simulink model "fengji"  (R2025a)
settings: Solver=VariableStepAuto  StartTime=0.0  StopTime=3  RelTol=1e-3
values from neighbouring files (symbols this model uses):
  A = pi * R^2    (= 6082.12337735)    [DFIG.m]    (also in Ref_and_Para.m)
  V = 0.9998    [Copy_2_of_wangce.m]    (also in Copy_2_of_wangceRef_and_Para.m; Copy_of_wangce.m; Copy_of_wangceRef_and_Para.m; DFIG.m)
undefined symbols (not defined in the file or in its folder): sigbuilder_block
libraries: slpidlib x6, spsabctodq0Lib x4, simulink x2, spsPLL3phLib x2, spsSVPWMGenerator2LevelLib x2, spsdq0toAlphaBetaZeroLib x2, spsUniversalBridgeLib x2, spsPower3phInstantaneousLib x1, spsSeriesRLCBranchLib x1, spsThreePhaseSeriesRLCBranchLib x1, spsThreePhaseVIMeasurementLib x1, spsThreePhaseSourceLib x1
settings Model: Creator=龙熠的本  LastModifiedBy=wz
settings SolverCC: AlgebraicLoopSolver=TrustRegion
settings DataIOCC: ReturnWorkspaceOutputs=off
settings DebuggingCC: UnconnectedInputMsg=warning  UnconnectedOutputMsg=warning  UnconnectedLineMsg=warning
settings ModelReferenceCC: EnableRefExpFcnMdlSchedulingChecks=on
settings RTWCC: GPUComputeCapability=3.5

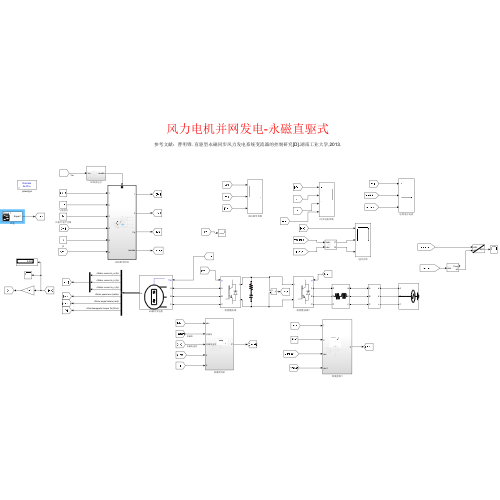
[thumbnail: Simulink's stored preview of the top-level diagram]
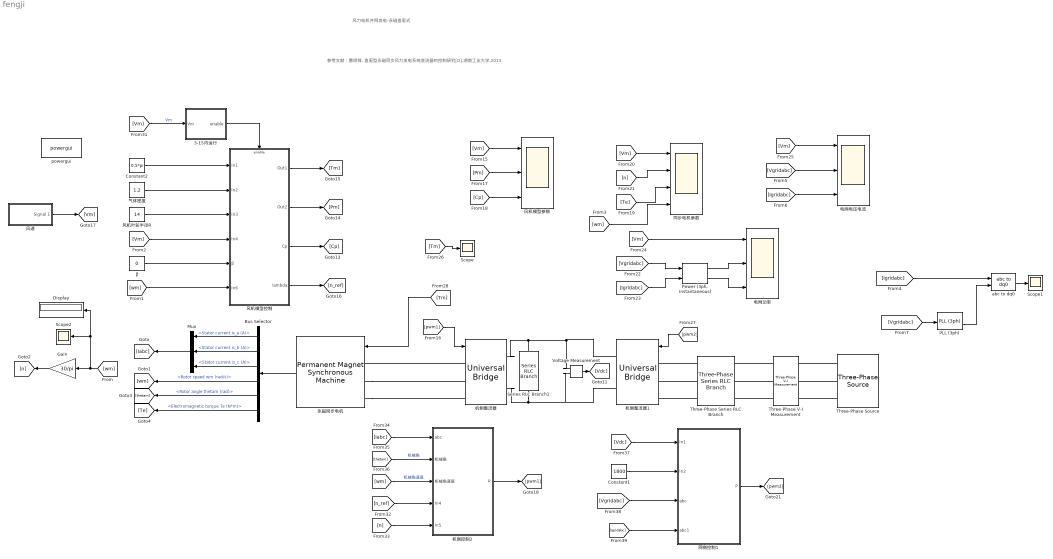
== system fengji ==
  note: 参考文献：曹明锋. 直驱型永磁同步风力发电系统变流器的控制研究[D].湖南工业大学,2013.
  note: 风力电机并网发电-永磁直驱式
  3-15内运行 : Subsystem
  Bus Selector : BusSelector  OutputSignals=Stator current is_a (A),Stator current is_b (A),Stator current is_c (A),Rotor speed wm (rad/s),Rotor angle thetam (rad),Electromagnetic torque Te (N*m)
  Constant1 : Constant  Value=1800
  Constant2 : Constant  Value=0.5*pi
  Display : Display
  Gain : Gain  Gain=30/pi
  Mux : Mux  Inputs=3
  PLL (3ph) : spsPLL3phLib/PLL (3ph)  Fmin=45  Par_Init=[0, 60]  ParK=[180, 3200, 1]  TcD=1e-4  MaxRateChangeFreq=12  FilterCutOffFreq=25  Ts=0  AGC=on
  "Power (3ph, Instantaneous)" : spsPower3phInstantaneousLib/Power (3ph, Instantaneous)
  Scope : Scope
      settings: ActiveDisplayYMinimum=-53568.9347809082  ActiveDisplayYMaximum=328.75957744243624  DataLoggingVariableName=ScopeData4
  Scope1 : Scope
      settings: ActiveDisplayYMinimum=-107.45342  ActiveDisplayYMaximum=357.3639
  Scope2 : Scope
      settings: DataLoggingVariableName=ScopeData9
  Series RLC Branch1 : spsSeriesRLCBranchLib/Series RLC Branch  LConnTagsString=__new0  RConnTagsString=__new0  BranchType=RC  Resistance=0.05  Inductance=1e-2  SetiL0=off  InitialCurrent=0  Capacitance=1e-3  Setx0=on  InitialVoltage=1800  Measurements=None
  Three-Phase Series RLC Branch : spsThreePhaseSeriesRLCBranchLib/Three-Phase Series RLC Branch  LConnTagsString=A|B|C  RConnTagsString=A|B|C  BranchType=RL  Resistance=0.05  Inductance=7e-3  Capacitance=1e-6  Measurements=None
  Three-Phase V-I Measurement : spsThreePhaseVIMeasurementLib/Three-Phase V-I Measurement  VoltageMeasurement=phase-to-ground  SetLabelV=on  LabelV=Vgridabc  Vpu=off  VpuLL=off  CurrentMeasurement=yes  SetLabelI=on  LabelI=Igridabc  Ipu=off  Pbase=100e6  Vbase=500e3  OutputType=Complex  PhasorSimulation=off  PSBequivalent=0
  Three-Phase Source : spsThreePhaseSourceLib/Three-Phase Source  InternalConnection=Yg  VoltagePhases=off  Voltage=690  PhaseAngle=0  Voltage_phases=[25e3 25e3 25e3]/sqrt(3)  PhaseAngles_phases=[0 -120 +120]  Frequency=50  NonIdealSource=off  SpecifyImpedance=off  Resistance=0.8929  Inductance=16.58e-3  ShortCircuitLevel=100e6  BaseVoltage=25e3  XRratio=7  BusType=swing  Pref=10e3  Qref=0  Prefabc=[10e3, 10e3, 10e3]  Qrefabc=[0, 0, 0]  Qmin=-inf  Qmax=inf
  Voltage Measurement : spsVoltageMeasurementLib/Voltage Measurement  PhasorSimulation=off  OutputType=Complex  PSBequivalent=0
  abc to dq0 : spsabctodq0Lib/abc to dq0  Alignment=90 degrees behind phase A axis
  powergui : sps_lib/powergui  Priority=1  SimulationMode=Discrete  SampleTime=2e-5  frequency=60  Iterations=50  frequencyindice=0  Pbase=100e6  ErrMax=1e-4  UnitsV=kV  UnitsW=MW  buscounter=0  FunctionMessages=off  echomessages=off  EnableUseOfTLC=off  CurrentSourceSwitches=off  DisableSnubberDevices=off  DisableRonSwitches=off  DisableVfSwitches=off  DisplayEquations=off  AutomaticDiscreteSolvers=off  SolverType=Tustin/Backward Euler (TBE)  Interpol=off  ExternalGateDelay=off  methode=off  Ts=100  x0status=blocks  SPID=on  SwTol=0  HookPort=off  NonlinearTolerance=1e-4  nMaxIteration=100  ContinueOnMaxIteration=off  RestoreLinks=warning  ResistiveCurrentMeasurement=off  Frange=[0:2:500]  Ylog=off  Xlog=on  ShowGrid=off  save=off  variable=ZData  structure=ScopeData3  ZoomFFT=off  StartTime=1.5  cycles=40  DisplayStyle=1  fundamental=50  FreqAxis=off  MaxFrequency=1000  frequencyindicesteady=1  RmsSteady=1  display=off
  β : Constant  Value=0
  同步电机参数 : Scope  NumInputPorts=4
      settings: ActiveDisplayYMinimum=7.5  ActiveDisplayYMaximum=12.5
  机侧控制2 : Subsystem
  机侧整流器 : spsUniversalBridgeLib/Universal Bridge  Arms=3  SnubberResistance=1e5  SnubberCapacitance=inf  Device=IGBT / Diodes  Ron=1e-3  Lon=0  ForwardVoltages="[  0  0  ]"  ForwardVoltage=0  GTOparameters=[ 10e-6 , 20e-6 ]  IGBTparameters=[ 1e-6 , 2e-6 ]  Measurements=None  Measurements_2=None  converterType=Rectifier
  机侧整流器1 : spsUniversalBridgeLib/Universal Bridge  Arms=3  SnubberResistance=1e5  SnubberCapacitance=inf  Device=IGBT / Diodes  Ron=1e-3  Lon=0  ForwardVoltages="[  0  0  ]"  ForwardVoltage=0  GTOparameters=[ 10e-6 , 20e-6 ]  IGBTparameters=[ 1e-6 , 2e-6 ]  Measurements=None  Measurements_2=None  converterType=Rectifier
  气体密度 : Constant  Value=1.2
  永磁同步电机 : spsPermanentMagnetSynchronousMachineLib/Permanent Magnet Synchronous Machine  NbPhases=3  FluxDistribution=Sinusoidal  RotorType=Round  MechanicalLoad=Torque Tm  PresetModel=No  ShowDetailedParameters=on  MeasurementBus=off  Resistance=0.025  Inductance=8.5e-3  dqInductances=[8.5e-3,8.5e-3]  La=0.0036  MachineConstant=Flux linkage established by magnets (V.s)  Flux=3.88889  VoltageCst=8464.3995  TorqueCst=70  Flat=120  Mechanical=[60 0.078 12]  PolePairs=4  InitialConditions=[0,0, 0,0]  InitialConditions5ph=[0 0 0 0 0 0]  RefAngle=90 degrees behind phase A axis (modified Park)  IterativeDiscreteModel=Trapezoidal non iterative  TsBlock=-1  TsPowergui=0
  电网功率 : Scope  NumInputPorts=3
      settings: ActiveDisplayYMinimum=2  ActiveDisplayYMaximum=22  DataLoggingVariableName=ScopeData2
  电网电压电流 : Scope  NumInputPorts=3
      settings: ActiveDisplayYMinimum=7.5  ActiveDisplayYMaximum=12.5  DataLoggingVariableName=ScopeData3
  网侧控制1 : Subsystem
  风机叶轮半径R : Constant  Value=14
  风机模型参数 : Scope  NumInputPorts=3
      settings: ActiveDisplayYMinimum=5.7582077  ActiveDisplayYMaximum=8.249088033333333
  风机模型控制 : Subsystem
  风速 : Subsystem  Tag=STV Subsys  LoadFcn=sigbuilder_block('load',[252.75 107.25 644.25 387.75 ]);  StartFcn=sigbuilder_block('start');  StopFcn=sigbuilder_block('stop');  ClipboardFcn=sigbuilder_block('clipboard');  mask(Sigbuilder block){tuvar=[0:10]}
      mask help: Simulink:masks:SigbuilderBlock_MD
      mask init:
      | if ~strcmp(get_param(bdroot(gcbh),'SimulationStatus'),'stopped') tuvar = sigbuilder_block('maskInit'); end
      settings: CopyFcn=sigbuilder_block('copy');  DeleteFcn=sigbuilder_block('delete');  ModelCloseFcn=sigbuilder_block('modelClose');  PreSaveFcn=sigbuilder_block('preSave');  PauseFcn=sigbuilder_block('pause');  ContinueFcn=sigbuilder_block('continue');  NameChangeFcn=sigbuilder_block('namechange');  OpenFcn=sigbuilder_block('open',[252.75 107.25 644.25 387.75 ]);  CloseFcn=sigbuilder_block('close');
      mask Display: plot(0, 0, 100, 100,[2, 2, 32, 32, 2], [68, 8, 8, 68, 68],[32, 2], [38, 38], [32, 19, 2],[53, 60, 44], [32, 17, 17, 2],[16, 16, 31, 31]);txt = getActiveGroup(gcbh);text(2, 100, txt,'verticalAlignment', 'top');
  wires:
  永磁同步电机/1 -> Bus Selector/1
  Bus Selector/2 -> Mux/2  "<Stator current is_b (A)>"
  Bus Selector/1 -> Mux/1  "<Stator current is_a (A)>"
  Bus Selector/3 -> Mux/3  "<Stator current is_c (A)>"
  Bus Selector/4 -> [wm]  "<Rotor speed wm (rad/s)>"
  Mux/1 -> [Iabc]
  Gain/1 -> [n]
  Bus Selector/5 -> [thetam]  "<Rotor angle thetam (rad)>"
  Bus Selector/6 -> [Te]  "<Electromagnetic torque Te (N*m)>"
  [wm] -> Display/1, Scope2/1, Gain/1
  [Tm] -> 永磁同步电机/1
  [pwm1] -> 机侧整流器/1
  [pwm2] -> 机侧整流器1/1
  [Vm] -> 风机模型参数/1
  [Pm] -> 风机模型参数/2
  [Cp] -> 风机模型参数/3
  [Vm] -> 同步电机参数/1
  [n] -> 同步电机参数/2
  [Te] -> 同步电机参数/3
  [Vgridabc] -> "Power (3ph, Instantaneous)"/1
  [Igridabc] -> "Power (3ph, Instantaneous)"/2
  "Power (3ph, Instantaneous)"/2 -> 电网功率/3
  "Power (3ph, Instantaneous)"/1 -> 电网功率/2
  [Vm] -> 电网功率/1
  [Vm] -> 电网电压电流/1
  [Vgridabc] -> 电网电压电流/2
  [Igridabc] -> 电网电压电流/3
  [Tm] -> Scope/1
  机侧控制2/1(P) -> [pwm1]
  [n] -> 机侧控制2/5(In5)
  [thetam] -> 机侧控制2/2(机械角)  "机械角"
  [Iabc] -> 机侧控制2/1(abc)
  [wm] -> 机侧控制2/3(机械角速度)  "机械角速度"
  [n_ref] -> 机侧控制2/4(In4)
  [Vgridabc] -> 网侧控制1/3(abc)
  网侧控制1/1(P) -> [pwm2]
  [Igridabc] -> 网侧控制1/4(abc1)
  Constant1/1 -> 网侧控制1/2(In2)
  [Vdc] -> 网侧控制1/1(In1)
  风速/1(Signal 1) -> [Vm]
  风机叶轮半径R/1 -> 风机模型控制/3(In3)
  Constant2/1 -> 风机模型控制/1(In1)
  风机模型控制/1(Out1) -> [Tm]
  风机模型控制/4(lambda) -> [n_ref]
  β/1 -> 风机模型控制/5(β)
  风机模型控制/3(Cp) -> [Cp]
  风机模型控制/2(Out2) -> [Pm]
  [wm] -> 风机模型控制/6(In6)
  气体密度/1 -> 风机模型控制/2(In2)
  3-15内运行/1(enable) -> 风机模型控制/Enable
  [Vm] -> 风机模型控制/4(In4)
  [Vm] -> 3-15内运行/1(Vm)  "Vm"
  Voltage Measurement/1 -> [Vdc]
  [wm] -> 同步电机参数/4
  [Vgridabc] -> PLL (3ph)/1
  [Igridabc] -> abc to dq0/1
  PLL (3ph)/2 -> abc to dq0/2
  abc to dq0/1 -> Scope1/1
  connections:
  机侧整流器/LConn1 -- 永磁同步电机/LConn1
  永磁同步电机/LConn2 -- 机侧整流器/LConn2
  永磁同步电机/LConn3 -- 机侧整流器/LConn3
  机侧整流器/RConn2 -- Voltage Measurement/LConn2 -- 机侧整流器1/RConn2 -- Series RLC Branch1/RConn1
  机侧整流器/RConn1 -- Series RLC Branch1/LConn1 -- 机侧整流器1/RConn1 -- Voltage Measurement/LConn1
  Three-Phase Series RLC Branch/LConn3 -- 机侧整流器1/LConn3
  Three-Phase Series RLC Branch/LConn2 -- 机侧整流器1/LConn2
  Three-Phase Series RLC Branch/LConn1 -- 机侧整流器1/LConn1
  Three-Phase V-I Measurement/LConn3 -- Three-Phase Series RLC Branch/RConn3
  Three-Phase V-I Measurement/LConn2 -- Three-Phase Series RLC Branch/RConn2
  Three-Phase V-I Measurement/LConn1 -- Three-Phase Series RLC Branch/RConn1
  Three-Phase Source/RConn3 -- Three-Phase V-I Measurement/RConn3
  Three-Phase Source/RConn2 -- Three-Phase V-I Measurement/RConn2
  Three-Phase Source/RConn1 -- Three-Phase V-I Measurement/RConn1

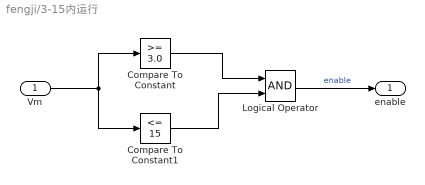
== system fengji/3-15内运行 ==
  Vm : Inport
  Compare To Constant : simulink/Logic and Bit Operations/Compare To Constant  relop=>=  const=3.0  OutDataTypeStr=boolean
  Compare To Constant1 : simulink/Logic and Bit Operations/Compare To Constant  relop=<=  const=15  OutDataTypeStr=boolean
  Logical Operator : Logic  AllPortsSameDT=off  OutDataTypeStr=boolean
  enable : Outport
  wires:
  Vm/1 -> Compare To Constant/1, Compare To Constant1/1
  Compare To Constant1/1 -> Logical Operator/2
  Logical Operator/1 -> enable/1  "enable"
  Compare To Constant/1 -> Logical Operator/1

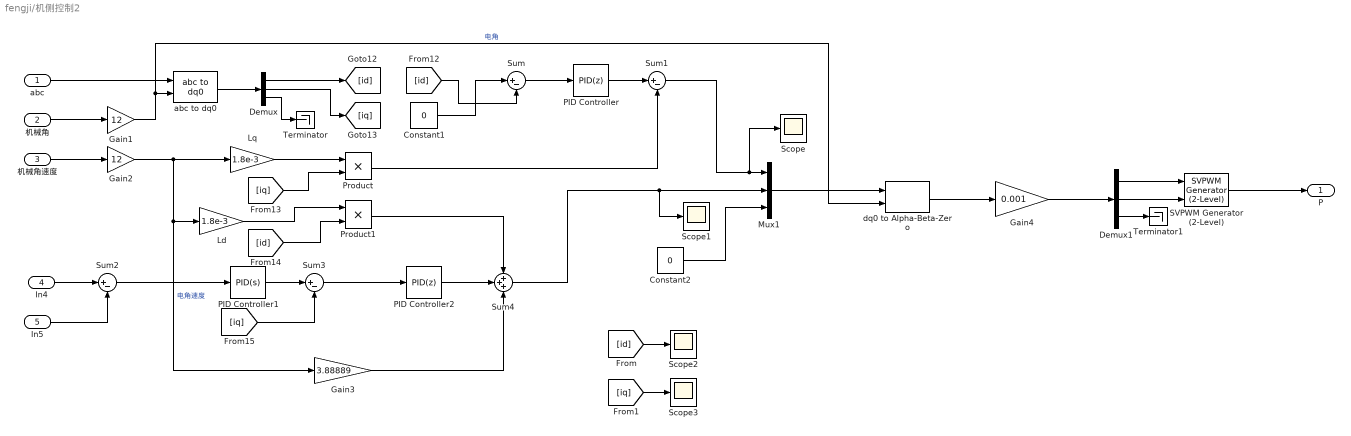
== system fengji/机侧控制2 ==
  abc : Inport
  机械角 : Inport  Port=2
  机械角速度 : Inport  Port=3
  In4 : Inport  Port=4
  In5 : Inport  Port=5
  Constant1 : Constant  Value=0
  Constant2 : Constant  Value=0
  Demux : Demux  Outputs=3
  Demux1 : Demux  Outputs=3
  Gain1 : Gain  Gain=12
  Gain2 : Gain  Gain=12
  Gain3 : Gain  Gain=3.88889
  Gain4 : Gain  Gain=0.001
  Ld : Gain  Gain=1.8e-3
  Lq : Gain  Gain=1.8e-3
  Mux1 : Mux  Inputs=3
  PID Controller : slpidlib/PID Controller  Controller=PID  Form=Parallel  TimeDomain=Discrete-time  UseExternalTs=off  SampleTime=-1  IntegratorMethod=Forward Euler  FilterMethod=Forward Euler  ControllerParametersSource=internal  P=1  I=12  UseKiTs=off  D=0  UseExternalDerivativeSource=off  N=100  UseFilter=on  TunerSelectOption=Transfer Function Based (PID Tuner App)  InitialConditionSource=internal  InitialConditionForIntegrator=0  InitialConditionForFilter=0  DifferentiatorICPrevScaledInput=0  ExternalReset=none  TrackingMode=off  Kt=1  LimitOutput=off  SatLimitsSource=internal  UpperSaturationLimit=inf  LowerSaturationLimit=-inf  LinearizeAsGain=on  AntiWindupMode=none  Kb=1  LimitIntegrator=off  UpperIntegratorSaturationLimit=inf  LowerIntegratorSaturationLimit=-inf  POutMin=[]  POutMax=[]  IOutMin=[]  IOutMax=[]  DOutMin=[]  DOutMax=[]  NOutMin=[]  NOutMax=[]  SumOutMin=[]  SumOutMax=[]  SaturationOutMin=[]  SaturationOutMax=[]  PParamMin=[]  PParamMax=[]  IParamMin=[]  IParamMax=[]  DParamMin=[]  DParamMax=[]  NParamMin=[]  NParamMax=[]  KbParamMin=[]  KbParamMax=[]  KtParamMin=[]  KtParamMax=[]  KbOutMin=[]  KbOutMax=[]  KtOutMin=[]  KtOutMax=[]  IntegratorOutMin=[]  IntegratorOutMax=[]  FilterOutMin=[]  FilterOutMax=[]  SumI1OutMin=[]  SumI1OutMax=[]  SumI2OutMin=[]  SumI2OutMax=[]  SumI3OutMin=[]  SumI3OutMax=[]  SumI4OutMin=[]  SumI4OutMax=[]  SumDOutMin=[]  SumDOutMax=[]  DifferentiatorOutMin=[]  DifferentiatorOutMax=[]  FilterDiffOutCoefMin=[]  FilterDiffOutCoefMax=[]  ReciprocalOutMin=[]  ReciprocalOutMax=[]  SumDenOutMin=[]  SumDenOutMax=[]  SumNumOutMin=[]  SumNumOutMax=[]  DivideOutMin=[]  DivideOutMax=[]  UdiffTsProdOutMin=[]  UdiffTsProdOutMax=[]  NTsProdOutMin=[]  NTsProdOutMax=[]  UintegralTsProdOutMin=[]  UintegralTsProdOutMax=[]  UngainTsProdOutMin=[]  UngainTsProdOutMax=[]  ClampingZeroOutDataTypeStr=Inherit: Inherit via back propagation  ClampingZeroOutMin=[]  ClampingZeroOutMax=[]  FilterDenConstantOutDataTypeStr=Inherit: Inherit via back propagation  FilterDenConstantOutMin=[]  FilterDenConstantOutMax=[]  PCopyOutDataTypeStr=Inherit: Inherit via back propagation  PCopyOutMin=[]  PCopyOutMax=[]  NCopyOutDataTypeStr=Inherit: Inherit via back propagation  NCopyOutMin=[]  NCopyOutMax=[]  IntegratorContinuousStateAttributes=''  IntegratorStateMustResolveToSignalObject=off  IntegratorRTWStateStorageClass=Auto  FilterContinuousStateAttributes=''  FilterStateMustResolveToSignalObject=off  FilterRTWStateStorageClass=Auto  ParallelPVariant=InternalParameters  IdealPVariant=Disabled  IVariant=InternalParameters  DVariant=InternalParameters  IntegratorVariant=Discrete  SatVariant=Disabled  AWVariant=Passthrough  PCopyVariant=Disabled  TRVariant=Disabled  FdbkBlocksVariant=Forward  IdealPFdbkVariant=Disabled  SatFdbkVariant=Disabled  DerivativeFilterVariant=ForwardEulerFilter  NVariant=InternalParameters  NCopyVariant=Disabled  FilterICVariant=InternalICsFilter  IntegratorICVariant=InternalICs  ExternalResetVariant=Disabled  TRSumVariant=Passthrough  SumFdbkVariant=Disabled  SumVariant=Sum_PID  TsampFilterVariant=InternalTs  TsampNgainVariant=Passthrough  TsampIntegralVariant=Disabled_SignalSpec  ExternalSaturationOutDataTypeStr=Inherit: Same as second input  DerivativeSourceVariant=ErrorSignal  PreIntVariant=InternalPreInt
  PID Controller1 : slpidlib/PID Controller  Controller=PID  Form=Parallel  TimeDomain=Continuous-time  UseExternalTs=off  SampleTime=-1  IntegratorMethod=Forward Euler  FilterMethod=Forward Euler  ControllerParametersSource=internal  P=10  I=220  UseKiTs=off  D=0  UseExternalDerivativeSource=off  N=100  UseFilter=on  TunerSelectOption=Transfer Function Based (PID Tuner App)  InitialConditionSource=internal  InitialConditionForIntegrator=0  InitialConditionForFilter=0  DifferentiatorICPrevScaledInput=0  ExternalReset=none  TrackingMode=off  Kt=1  LimitOutput=off  SatLimitsSource=internal  UpperSaturationLimit=inf  LowerSaturationLimit=-inf  LinearizeAsGain=on  AntiWindupMode=none  Kb=1  LimitIntegrator=off  UpperIntegratorSaturationLimit=inf  LowerIntegratorSaturationLimit=-inf  POutMin=[]  POutMax=[]  IOutMin=[]  IOutMax=[]  DOutMin=[]  DOutMax=[]  NOutMin=[]  NOutMax=[]  SumOutMin=[]  SumOutMax=[]  SaturationOutMin=[]  SaturationOutMax=[]  PParamMin=[]  PParamMax=[]  IParamMin=[]  IParamMax=[]  DParamMin=[]  DParamMax=[]  NParamMin=[]  NParamMax=[]  KbParamMin=[]  KbParamMax=[]  KtParamMin=[]  KtParamMax=[]  KbOutMin=[]  KbOutMax=[]  KtOutMin=[]  KtOutMax=[]  IntegratorOutMin=[]  IntegratorOutMax=[]  FilterOutMin=[]  FilterOutMax=[]  SumI1OutMin=[]  SumI1OutMax=[]  SumI2OutMin=[]  SumI2OutMax=[]  SumI3OutMin=[]  SumI3OutMax=[]  SumI4OutMin=[]  SumI4OutMax=[]  SumDOutMin=[]  SumDOutMax=[]  DifferentiatorOutMin=[]  DifferentiatorOutMax=[]  FilterDiffOutCoefMin=[]  FilterDiffOutCoefMax=[]  ReciprocalOutMin=[]  ReciprocalOutMax=[]  SumDenOutMin=[]  SumDenOutMax=[]  SumNumOutMin=[]  SumNumOutMax=[]  DivideOutMin=[]  DivideOutMax=[]  UdiffTsProdOutMin=[]  UdiffTsProdOutMax=[]  NTsProdOutMin=[]  NTsProdOutMax=[]  UintegralTsProdOutMin=[]  UintegralTsProdOutMax=[]  UngainTsProdOutMin=[]  UngainTsProdOutMax=[]  ClampingZeroOutDataTypeStr=Inherit: Inherit via back propagation  ClampingZeroOutMin=[]  ClampingZeroOutMax=[]  FilterDenConstantOutDataTypeStr=Inherit: Inherit via back propagation  FilterDenConstantOutMin=[]  FilterDenConstantOutMax=[]  PCopyOutDataTypeStr=Inherit: Inherit via back propagation  PCopyOutMin=[]  PCopyOutMax=[]  NCopyOutDataTypeStr=Inherit: Inherit via back propagation  NCopyOutMin=[]  NCopyOutMax=[]  IntegratorContinuousStateAttributes=''  IntegratorStateMustResolveToSignalObject=off  IntegratorRTWStateStorageClass=Auto  FilterContinuousStateAttributes=''  FilterStateMustResolveToSignalObject=off  FilterRTWStateStorageClass=Auto  ParallelPVariant=InternalParameters  IdealPVariant=Disabled  IVariant=InternalParameters  DVariant=InternalParameters  IntegratorVariant=Continuous  SatVariant=Disabled  AWVariant=Passthrough  PCopyVariant=Disabled  TRVariant=Disabled  FdbkBlocksVariant=Forward  IdealPFdbkVariant=Disabled  SatFdbkVariant=Disabled  DerivativeFilterVariant=ContFilter  NVariant=InternalParameters  NCopyVariant=Disabled  FilterICVariant=InternalICsFilter  IntegratorICVariant=InternalICs  ExternalResetVariant=Disabled  TRSumVariant=Passthrough  SumFdbkVariant=Disabled  SumVariant=Sum_PID  TsampFilterVariant=InternalTs  TsampNgainVariant=Passthrough  TsampIntegralVariant=Disabled_SignalSpec  ExternalSaturationOutDataTypeStr=Inherit: Same as second input  DerivativeSourceVariant=ErrorSignal  PreIntVariant=InternalPreInt
  PID Controller2 : slpidlib/PID Controller  Controller=PID  Form=Parallel  TimeDomain=Discrete-time  UseExternalTs=off  SampleTime=-1  IntegratorMethod=Forward Euler  FilterMethod=Forward Euler  ControllerParametersSource=internal  P=1  I=12  UseKiTs=off  D=0  UseExternalDerivativeSource=off  N=100  UseFilter=on  TunerSelectOption=Transfer Function Based (PID Tuner App)  InitialConditionSource=internal  InitialConditionForIntegrator=0  InitialConditionForFilter=0  DifferentiatorICPrevScaledInput=0  ExternalReset=none  TrackingMode=off  Kt=1  LimitOutput=off  SatLimitsSource=internal  UpperSaturationLimit=inf  LowerSaturationLimit=-inf  LinearizeAsGain=on  AntiWindupMode=none  Kb=1  LimitIntegrator=off  UpperIntegratorSaturationLimit=inf  LowerIntegratorSaturationLimit=-inf  POutMin=[]  POutMax=[]  IOutMin=[]  IOutMax=[]  DOutMin=[]  DOutMax=[]  NOutMin=[]  NOutMax=[]  SumOutMin=[]  SumOutMax=[]  SaturationOutMin=[]  SaturationOutMax=[]  PParamMin=[]  PParamMax=[]  IParamMin=[]  IParamMax=[]  DParamMin=[]  DParamMax=[]  NParamMin=[]  NParamMax=[]  KbParamMin=[]  KbParamMax=[]  KtParamMin=[]  KtParamMax=[]  KbOutMin=[]  KbOutMax=[]  KtOutMin=[]  KtOutMax=[]  IntegratorOutMin=[]  IntegratorOutMax=[]  FilterOutMin=[]  FilterOutMax=[]  SumI1OutMin=[]  SumI1OutMax=[]  SumI2OutMin=[]  SumI2OutMax=[]  SumI3OutMin=[]  SumI3OutMax=[]  SumI4OutMin=[]  SumI4OutMax=[]  SumDOutMin=[]  SumDOutMax=[]  DifferentiatorOutMin=[]  DifferentiatorOutMax=[]  FilterDiffOutCoefMin=[]  FilterDiffOutCoefMax=[]  ReciprocalOutMin=[]  ReciprocalOutMax=[]  SumDenOutMin=[]  SumDenOutMax=[]  SumNumOutMin=[]  SumNumOutMax=[]  DivideOutMin=[]  DivideOutMax=[]  UdiffTsProdOutMin=[]  UdiffTsProdOutMax=[]  NTsProdOutMin=[]  NTsProdOutMax=[]  UintegralTsProdOutMin=[]  UintegralTsProdOutMax=[]  UngainTsProdOutMin=[]  UngainTsProdOutMax=[]  ClampingZeroOutDataTypeStr=Inherit: Inherit via back propagation  ClampingZeroOutMin=[]  ClampingZeroOutMax=[]  FilterDenConstantOutDataTypeStr=Inherit: Inherit via back propagation  FilterDenConstantOutMin=[]  FilterDenConstantOutMax=[]  PCopyOutDataTypeStr=Inherit: Inherit via back propagation  PCopyOutMin=[]  PCopyOutMax=[]  NCopyOutDataTypeStr=Inherit: Inherit via back propagation  NCopyOutMin=[]  NCopyOutMax=[]  IntegratorContinuousStateAttributes=''  IntegratorStateMustResolveToSignalObject=off  IntegratorRTWStateStorageClass=Auto  FilterContinuousStateAttributes=''  FilterStateMustResolveToSignalObject=off  FilterRTWStateStorageClass=Auto  ParallelPVariant=InternalParameters  IdealPVariant=Disabled  IVariant=InternalParameters  DVariant=InternalParameters  IntegratorVariant=Discrete  SatVariant=Disabled  AWVariant=Passthrough  PCopyVariant=Disabled  TRVariant=Disabled  FdbkBlocksVariant=Forward  IdealPFdbkVariant=Disabled  SatFdbkVariant=Disabled  DerivativeFilterVariant=ForwardEulerFilter  NVariant=InternalParameters  NCopyVariant=Disabled  FilterICVariant=InternalICsFilter  IntegratorICVariant=InternalICs  ExternalResetVariant=Disabled  TRSumVariant=Passthrough  SumFdbkVariant=Disabled  SumVariant=Sum_PID  TsampFilterVariant=InternalTs  TsampNgainVariant=Passthrough  TsampIntegralVariant=Disabled_SignalSpec  ExternalSaturationOutDataTypeStr=Inherit: Same as second input  DerivativeSourceVariant=ErrorSignal  PreIntVariant=InternalPreInt
  Product : Product
  Product1 : Product
  SVPWM Generator (2-Level) : spsSVPWMGenerator2LevelLib/SVPWM Generator (2-Level)  InputType=alpha-beta components  SwitchingPattern=Pattern #1  Fc=3e3  ParUref=[0.8 -30 50]  Ts=0
  Scope{,1..3} (4 alike) : Scope
      Scope settings: ActiveDisplayYMinimum=-77.246328045068424  ActiveDisplayYMaximum=250.40861499738187  DataLoggingVariableName=ScopeData5
      Scope1 settings: ActiveDisplayYMinimum=51.447457334702889  ActiveDisplayYMaximum=486.78738885568737  DataLoggingVariableName=ScopeData6
      Scope2 settings: ActiveDisplayYMinimum=-70.304855275250532  ActiveDisplayYMaximum=40.582386040383945  DataLoggingVariableName=ScopeData7
      Scope3 settings: ActiveDisplayYMinimum=-769.28635625376307  ActiveDisplayYMaximum=430.28722806240035  DataLoggingVariableName=ScopeData8
  Sum{,1..3} (4 alike) : Sum  Inputs=|+-
  Sum4 : Sum  Inputs=+++
  Terminator : Terminator
  Terminator1 : Terminator
  abc to dq0 : spsabctodq0Lib/abc to dq0  Alignment=90 degrees behind phase A axis
  dq0 to Alpha-Beta-Zero : spsdq0toAlphaBetaZeroLib/dq0 to Alpha-Beta-Zero  Alignment=90 degrees behind phase A axis
  P : Outport
  wires:
  Sum4/1 -> Scope1/1, Mux1/2
  PID Controller1/1 -> Sum3/1
  Demux/2 -> [iq]
  Sum1/1 -> Scope/1, Mux1/1
  Demux/3 -> Terminator/1
  dq0 to Alpha-Beta-Zero/1 -> Gain4/1
  Demux/1 -> [id]
  SVPWM Generator (2-Level)/1 -> P/1
  [iq] -> Product/2
  Lq/1 -> Product/1
  [iq] -> Sum3/2
  [id] -> Product1/2
  Demux1/2 -> SVPWM Generator (2-Level)/2
  Sum/1 -> PID Controller/1
  Product/1 -> Sum1/2
  Gain1/1 -> dq0 to Alpha-Beta-Zero/2, abc to dq0/2  "电角"
  In4/1 -> Sum2/1
  Demux1/3 -> Terminator1/1
  Constant2/1 -> Mux1/3
  PID Controller2/1 -> Sum4/2
  abc to dq0/1 -> Demux/1
  Sum3/1 -> PID Controller2/1
  PID Controller/1 -> Sum1/1
  In5/1 -> Sum2/2
  Gain2/1 -> Gain3/1, Ld/1, Lq/1  "电角速度"
  Sum2/1 -> PID Controller1/1
  Ld/1 -> Product1/1
  Mux1/1 -> dq0 to Alpha-Beta-Zero/1
  机械角/1 -> Gain1/1
  机械角速度/1 -> Gain2/1
  Product1/1 -> Sum4/1
  Demux1/1 -> SVPWM Generator (2-Level)/1
  Gain3/1 -> Sum4/3
  Gain4/1 -> Demux1/1
  abc/1 -> abc to dq0/1
  Constant1/1 -> Sum/1
  [id] -> Sum/2
  [id] -> Scope2/1
  [iq] -> Scope3/1

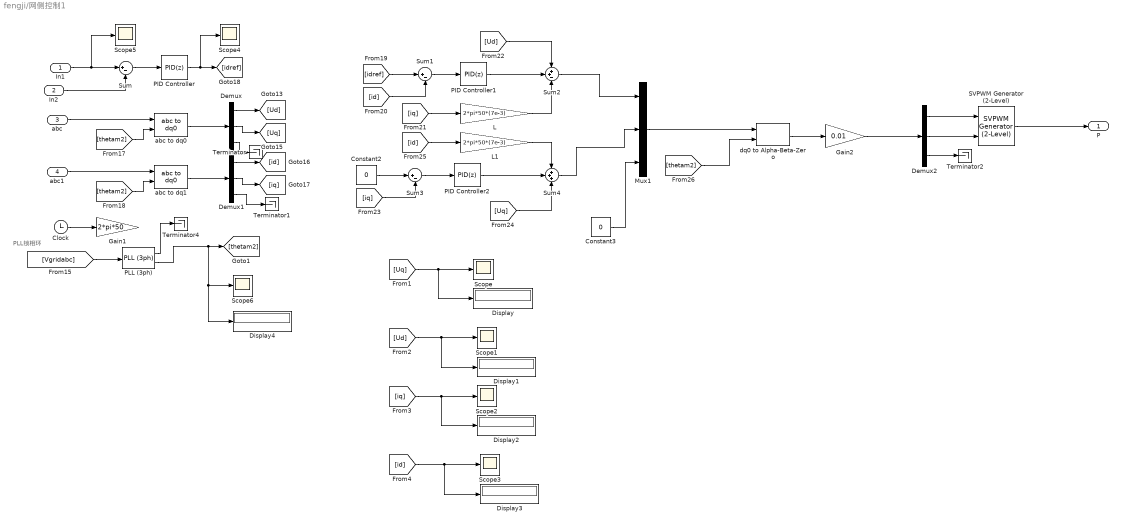
== system fengji/网侧控制1 ==
  note: PLL锁相环
  In1 : Inport
  In2 : Inport  Port=2
  abc : Inport  Port=3
  abc1 : Inport  Port=4
  Clock : Clock
  Constant2 : Constant  Value=0
  Constant3 : Constant  Value=0
  Demux : Demux  Outputs=3
  Demux1 : Demux  Outputs=3
  Demux2 : Demux  Outputs=3
  Display{,1..4} (5 alike) : Display
  Gain1 : Gain  Gain=2*pi*50
  Gain2 : Gain  Gain=0.01
  L : Gain  Gain=2*pi*50*(7e-3)
  L1 : Gain  Gain=2*pi*50*(7e-3)
  Mux1 : Mux  Inputs=3
  PID Controller : slpidlib/PID Controller  Controller=PID  Form=Parallel  TimeDomain=Discrete-time  UseExternalTs=off  SampleTime=-1  IntegratorMethod=Forward Euler  FilterMethod=Forward Euler  ControllerParametersSource=internal  P=1  I=10  UseKiTs=off  D=0  UseExternalDerivativeSource=off  N=100  UseFilter=on  TunerSelectOption=Transfer Function Based (PID Tuner App)  InitialConditionSource=internal  InitialConditionForIntegrator=0  InitialConditionForFilter=0  DifferentiatorICPrevScaledInput=0  ExternalReset=none  TrackingMode=off  Kt=1  LimitOutput=off  SatLimitsSource=internal  UpperSaturationLimit=inf  LowerSaturationLimit=-inf  LinearizeAsGain=on  AntiWindupMode=none  Kb=1  LimitIntegrator=off  UpperIntegratorSaturationLimit=inf  LowerIntegratorSaturationLimit=-inf  POutMin=[]  POutMax=[]  IOutMin=[]  IOutMax=[]  DOutMin=[]  DOutMax=[]  NOutMin=[]  NOutMax=[]  SumOutMin=[]  SumOutMax=[]  SaturationOutMin=[]  SaturationOutMax=[]  PParamMin=[]  PParamMax=[]  IParamMin=[]  IParamMax=[]  DParamMin=[]  DParamMax=[]  NParamMin=[]  NParamMax=[]  KbParamMin=[]  KbParamMax=[]  KtParamMin=[]  KtParamMax=[]  KbOutMin=[]  KbOutMax=[]  KtOutMin=[]  KtOutMax=[]  IntegratorOutMin=[]  IntegratorOutMax=[]  FilterOutMin=[]  FilterOutMax=[]  SumI1OutMin=[]  SumI1OutMax=[]  SumI2OutMin=[]  SumI2OutMax=[]  SumI3OutMin=[]  SumI3OutMax=[]  SumI4OutMin=[]  SumI4OutMax=[]  SumDOutMin=[]  SumDOutMax=[]  DifferentiatorOutMin=[]  DifferentiatorOutMax=[]  FilterDiffOutCoefMin=[]  FilterDiffOutCoefMax=[]  ReciprocalOutMin=[]  ReciprocalOutMax=[]  SumDenOutMin=[]  SumDenOutMax=[]  SumNumOutMin=[]  SumNumOutMax=[]  DivideOutMin=[]  DivideOutMax=[]  UdiffTsProdOutMin=[]  UdiffTsProdOutMax=[]  NTsProdOutMin=[]  NTsProdOutMax=[]  UintegralTsProdOutMin=[]  UintegralTsProdOutMax=[]  UngainTsProdOutMin=[]  UngainTsProdOutMax=[]  ClampingZeroOutDataTypeStr=Inherit: Inherit via back propagation  ClampingZeroOutMin=[]  ClampingZeroOutMax=[]  FilterDenConstantOutDataTypeStr=Inherit: Inherit via back propagation  FilterDenConstantOutMin=[]  FilterDenConstantOutMax=[]  PCopyOutDataTypeStr=Inherit: Inherit via back propagation  PCopyOutMin=[]  PCopyOutMax=[]  NCopyOutDataTypeStr=Inherit: Inherit via back propagation  NCopyOutMin=[]  NCopyOutMax=[]  IntegratorContinuousStateAttributes=''  IntegratorStateMustResolveToSignalObject=off  IntegratorRTWStateStorageClass=Auto  FilterContinuousStateAttributes=''  FilterStateMustResolveToSignalObject=off  FilterRTWStateStorageClass=Auto  ParallelPVariant=InternalParameters  IdealPVariant=Disabled  IVariant=InternalParameters  DVariant=InternalParameters  IntegratorVariant=Discrete  SatVariant=Disabled  AWVariant=Passthrough  PCopyVariant=Disabled  TRVariant=Disabled  FdbkBlocksVariant=Forward  IdealPFdbkVariant=Disabled  SatFdbkVariant=Disabled  DerivativeFilterVariant=ForwardEulerFilter  NVariant=InternalParameters  NCopyVariant=Disabled  FilterICVariant=InternalICsFilter  IntegratorICVariant=InternalICs  ExternalResetVariant=Disabled  TRSumVariant=Passthrough  SumFdbkVariant=Disabled  SumVariant=Sum_PID  TsampFilterVariant=InternalTs  TsampNgainVariant=Passthrough  TsampIntegralVariant=Disabled_SignalSpec  ExternalSaturationOutDataTypeStr=Inherit: Same as second input  DerivativeSourceVariant=ErrorSignal  PreIntVariant=InternalPreInt
  PID Controller1 : slpidlib/PID Controller  Controller=PID  Form=Parallel  TimeDomain=Discrete-time  UseExternalTs=off  SampleTime=-1  IntegratorMethod=Forward Euler  FilterMethod=Forward Euler  ControllerParametersSource=internal  P=1  I=15  UseKiTs=off  D=0  UseExternalDerivativeSource=off  N=100  UseFilter=on  TunerSelectOption=Transfer Function Based (PID Tuner App)  InitialConditionSource=internal  InitialConditionForIntegrator=0  InitialConditionForFilter=0  DifferentiatorICPrevScaledInput=0  ExternalReset=none  TrackingMode=off  Kt=1  LimitOutput=off  SatLimitsSource=internal  UpperSaturationLimit=inf  LowerSaturationLimit=-inf  LinearizeAsGain=on  AntiWindupMode=none  Kb=1  LimitIntegrator=off  UpperIntegratorSaturationLimit=inf  LowerIntegratorSaturationLimit=-inf  POutMin=[]  POutMax=[]  IOutMin=[]  IOutMax=[]  DOutMin=[]  DOutMax=[]  NOutMin=[]  NOutMax=[]  SumOutMin=[]  SumOutMax=[]  SaturationOutMin=[]  SaturationOutMax=[]  PParamMin=[]  PParamMax=[]  IParamMin=[]  IParamMax=[]  DParamMin=[]  DParamMax=[]  NParamMin=[]  NParamMax=[]  KbParamMin=[]  KbParamMax=[]  KtParamMin=[]  KtParamMax=[]  KbOutMin=[]  KbOutMax=[]  KtOutMin=[]  KtOutMax=[]  IntegratorOutMin=[]  IntegratorOutMax=[]  FilterOutMin=[]  FilterOutMax=[]  SumI1OutMin=[]  SumI1OutMax=[]  SumI2OutMin=[]  SumI2OutMax=[]  SumI3OutMin=[]  SumI3OutMax=[]  SumI4OutMin=[]  SumI4OutMax=[]  SumDOutMin=[]  SumDOutMax=[]  DifferentiatorOutMin=[]  DifferentiatorOutMax=[]  FilterDiffOutCoefMin=[]  FilterDiffOutCoefMax=[]  ReciprocalOutMin=[]  ReciprocalOutMax=[]  SumDenOutMin=[]  SumDenOutMax=[]  SumNumOutMin=[]  SumNumOutMax=[]  DivideOutMin=[]  DivideOutMax=[]  UdiffTsProdOutMin=[]  UdiffTsProdOutMax=[]  NTsProdOutMin=[]  NTsProdOutMax=[]  UintegralTsProdOutMin=[]  UintegralTsProdOutMax=[]  UngainTsProdOutMin=[]  UngainTsProdOutMax=[]  ClampingZeroOutDataTypeStr=Inherit: Inherit via back propagation  ClampingZeroOutMin=[]  ClampingZeroOutMax=[]  FilterDenConstantOutDataTypeStr=Inherit: Inherit via back propagation  FilterDenConstantOutMin=[]  FilterDenConstantOutMax=[]  PCopyOutDataTypeStr=Inherit: Inherit via back propagation  PCopyOutMin=[]  PCopyOutMax=[]  NCopyOutDataTypeStr=Inherit: Inherit via back propagation  NCopyOutMin=[]  NCopyOutMax=[]  IntegratorContinuousStateAttributes=''  IntegratorStateMustResolveToSignalObject=off  IntegratorRTWStateStorageClass=Auto  FilterContinuousStateAttributes=''  FilterStateMustResolveToSignalObject=off  FilterRTWStateStorageClass=Auto  ParallelPVariant=InternalParameters  IdealPVariant=Disabled  IVariant=InternalParameters  DVariant=InternalParameters  IntegratorVariant=Discrete  SatVariant=Disabled  AWVariant=Passthrough  PCopyVariant=Disabled  TRVariant=Disabled  FdbkBlocksVariant=Forward  IdealPFdbkVariant=Disabled  SatFdbkVariant=Disabled  DerivativeFilterVariant=ForwardEulerFilter  NVariant=InternalParameters  NCopyVariant=Disabled  FilterICVariant=InternalICsFilter  IntegratorICVariant=InternalICs  ExternalResetVariant=Disabled  TRSumVariant=Passthrough  SumFdbkVariant=Disabled  SumVariant=Sum_PID  TsampFilterVariant=InternalTs  TsampNgainVariant=Passthrough  TsampIntegralVariant=Disabled_SignalSpec  ExternalSaturationOutDataTypeStr=Inherit: Same as second input  DerivativeSourceVariant=ErrorSignal  PreIntVariant=InternalPreInt
  PID Controller2 : slpidlib/PID Controller  Controller=PID  Form=Parallel  TimeDomain=Discrete-time  UseExternalTs=off  SampleTime=-1  IntegratorMethod=Forward Euler  FilterMethod=Forward Euler  ControllerParametersSource=internal  P=1  I=15  UseKiTs=off  D=0  UseExternalDerivativeSource=off  N=100  UseFilter=on  TunerSelectOption=Transfer Function Based (PID Tuner App)  InitialConditionSource=internal  InitialConditionForIntegrator=0  InitialConditionForFilter=0  DifferentiatorICPrevScaledInput=0  ExternalReset=none  TrackingMode=off  Kt=1  LimitOutput=off  SatLimitsSource=internal  UpperSaturationLimit=inf  LowerSaturationLimit=-inf  LinearizeAsGain=on  AntiWindupMode=none  Kb=1  LimitIntegrator=off  UpperIntegratorSaturationLimit=inf  LowerIntegratorSaturationLimit=-inf  POutMin=[]  POutMax=[]  IOutMin=[]  IOutMax=[]  DOutMin=[]  DOutMax=[]  NOutMin=[]  NOutMax=[]  SumOutMin=[]  SumOutMax=[]  SaturationOutMin=[]  SaturationOutMax=[]  PParamMin=[]  PParamMax=[]  IParamMin=[]  IParamMax=[]  DParamMin=[]  DParamMax=[]  NParamMin=[]  NParamMax=[]  KbParamMin=[]  KbParamMax=[]  KtParamMin=[]  KtParamMax=[]  KbOutMin=[]  KbOutMax=[]  KtOutMin=[]  KtOutMax=[]  IntegratorOutMin=[]  IntegratorOutMax=[]  FilterOutMin=[]  FilterOutMax=[]  SumI1OutMin=[]  SumI1OutMax=[]  SumI2OutMin=[]  SumI2OutMax=[]  SumI3OutMin=[]  SumI3OutMax=[]  SumI4OutMin=[]  SumI4OutMax=[]  SumDOutMin=[]  SumDOutMax=[]  DifferentiatorOutMin=[]  DifferentiatorOutMax=[]  FilterDiffOutCoefMin=[]  FilterDiffOutCoefMax=[]  ReciprocalOutMin=[]  ReciprocalOutMax=[]  SumDenOutMin=[]  SumDenOutMax=[]  SumNumOutMin=[]  SumNumOutMax=[]  DivideOutMin=[]  DivideOutMax=[]  UdiffTsProdOutMin=[]  UdiffTsProdOutMax=[]  NTsProdOutMin=[]  NTsProdOutMax=[]  UintegralTsProdOutMin=[]  UintegralTsProdOutMax=[]  UngainTsProdOutMin=[]  UngainTsProdOutMax=[]  ClampingZeroOutDataTypeStr=Inherit: Inherit via back propagation  ClampingZeroOutMin=[]  ClampingZeroOutMax=[]  FilterDenConstantOutDataTypeStr=Inherit: Inherit via back propagation  FilterDenConstantOutMin=[]  FilterDenConstantOutMax=[]  PCopyOutDataTypeStr=Inherit: Inherit via back propagation  PCopyOutMin=[]  PCopyOutMax=[]  NCopyOutDataTypeStr=Inherit: Inherit via back propagation  NCopyOutMin=[]  NCopyOutMax=[]  IntegratorContinuousStateAttributes=''  IntegratorStateMustResolveToSignalObject=off  IntegratorRTWStateStorageClass=Auto  FilterContinuousStateAttributes=''  FilterStateMustResolveToSignalObject=off  FilterRTWStateStorageClass=Auto  ParallelPVariant=InternalParameters  IdealPVariant=Disabled  IVariant=InternalParameters  DVariant=InternalParameters  IntegratorVariant=Discrete  SatVariant=Disabled  AWVariant=Passthrough  PCopyVariant=Disabled  TRVariant=Disabled  FdbkBlocksVariant=Forward  IdealPFdbkVariant=Disabled  SatFdbkVariant=Disabled  DerivativeFilterVariant=ForwardEulerFilter  NVariant=InternalParameters  NCopyVariant=Disabled  FilterICVariant=InternalICsFilter  IntegratorICVariant=InternalICs  ExternalResetVariant=Disabled  TRSumVariant=Passthrough  SumFdbkVariant=Disabled  SumVariant=Sum_PID  TsampFilterVariant=InternalTs  TsampNgainVariant=Passthrough  TsampIntegralVariant=Disabled_SignalSpec  ExternalSaturationOutDataTypeStr=Inherit: Same as second input  DerivativeSourceVariant=ErrorSignal  PreIntVariant=InternalPreInt
  PLL (3ph) : spsPLL3phLib/PLL (3ph)  Fmin=45  Par_Init=[0, 50]  ParK=[180, 3200, 1]  TcD=1e-4  MaxRateChangeFreq=12  FilterCutOffFreq=25  Ts=0  AGC=on
  SVPWM Generator (2-Level) : spsSVPWMGenerator2LevelLib/SVPWM Generator (2-Level)  InputType=alpha-beta components  SwitchingPattern=Pattern #1  Fc=3000  ParUref=[0.8 -30 50]  Ts=0
  Scope{,1..6} (7 alike) : Scope
      Scope settings: ActiveDisplayYMinimum=-4.34345536667807  ActiveDisplayYMaximum=3.6929558988105935  DataLoggingVariableName=ScopeData10
      Scope1 settings: ActiveDisplayYMinimum=563.37013006275  ActiveDisplayYMaximum=563.38403092650674  DataLoggingVariableName=ScopeData11
      Scope2 settings: ActiveDisplayYMinimum=-203.1682368264394  ActiveDisplayYMaximum=403.27940369592733  DataLoggingVariableName=ScopeData12
      Scope3 settings: ActiveDisplayYMinimum=-661.11803433014575  ActiveDisplayYMaximum=608.254667322305  DataLoggingVariableName=ScopeData13
      Scope4 settings: ActiveDisplayYMinimum=-1055.4396971227802  ActiveDisplayYMaximum=1429.5603673337337  DataLoggingVariableName=ScopeData14
      Scope5 settings: ActiveDisplayYMinimum=806.5413726592958  ActiveDisplayYMaximum=3282.30252742951  DataLoggingVariableName=ScopeData15
      Scope6 settings: ActiveDisplayYMinimum=-0.785398163397448  ActiveDisplayYMaximum=7.0685834705770336  DataLoggingVariableName=ScopeData16
  Sum : Sum  Inputs=|+-
  Sum1 : Sum  Inputs=|+-
  Sum2 : Sum  Inputs=++-
  Sum3 : Sum  Inputs=|+-
  Sum4 : Sum  Inputs=+++
  Terminator{,1..2,4} (4 alike) : Terminator
  abc to dq0 : spsabctodq0Lib/abc to dq0  Alignment=90 degrees behind phase A axis
  abc to dq1 : spsabctodq0Lib/abc to dq0  Alignment=90 degrees behind phase A axis
  dq0 to Alpha-Beta-Zero : spsdq0toAlphaBetaZeroLib/dq0 to Alpha-Beta-Zero  Alignment=90 degrees behind phase A axis
  P : Outport
  wires:
  [thetam2] -> abc to dq1/2
  [id] -> Sum1/2
  abc to dq1/1 -> Demux1/1
  PID Controller/1 -> Scope4/1, [idref]
  Gain2/1 -> Demux2/1
  [thetam2] -> abc to dq0/2
  abc1/1 -> abc to dq1/1
  Sum4/1 -> Mux1/2
  [iq] -> Sum3/2
  abc to dq0/1 -> Demux/1
  Demux1/3 -> Terminator1/1
  Demux1/2 -> [iq]
  Constant2/1 -> Sum3/1
  Demux1/1 -> [id]
  PID Controller2/1 -> Sum4/2
  Demux2/1 -> SVPWM Generator (2-Level)/1
  L1/1 -> Sum4/1
  Demux/1 -> [Ud]
  SVPWM Generator (2-Level)/1 -> P/1
  Demux/3 -> Terminator/1
  [Vgridabc] -> PLL (3ph)/1
  Demux2/2 -> SVPWM Generator (2-Level)/2
  Demux/2 -> [Uq]
  PID Controller1/1 -> Sum2/2
  Sum1/1 -> PID Controller1/1
  L/1 -> Sum2/3
  Clock/1 -> Gain1/1
  Sum3/1 -> PID Controller2/1
  Sum/1 -> PID Controller/1
  Demux2/3 -> Terminator2/1
  Mux1/1 -> dq0 to Alpha-Beta-Zero/1
  dq0 to Alpha-Beta-Zero/1 -> Gain2/1
  [Ud] -> Sum2/1
  [iq] -> L/1
  In2/1 -> Sum/2
  [thetam2] -> dq0 to Alpha-Beta-Zero/2
  abc/1 -> abc to dq0/1
  [Uq] -> Sum4/3
  [idref] -> Sum1/1
  [id] -> L1/1
  In1/1 -> Scope5/1, Sum/1
  PLL (3ph)/2 -> Display4/1, Scope6/1, [thetam2]
  Constant3/1 -> Mux1/3
  Sum2/1 -> Mux1/1
  [Uq] -> Display/1, Scope/1
  [Ud] -> Scope1/1, Display1/1
  [id] -> Display3/1, Scope3/1
  [iq] -> Scope2/1, Display2/1
  PLL (3ph)/1 -> Terminator4/1

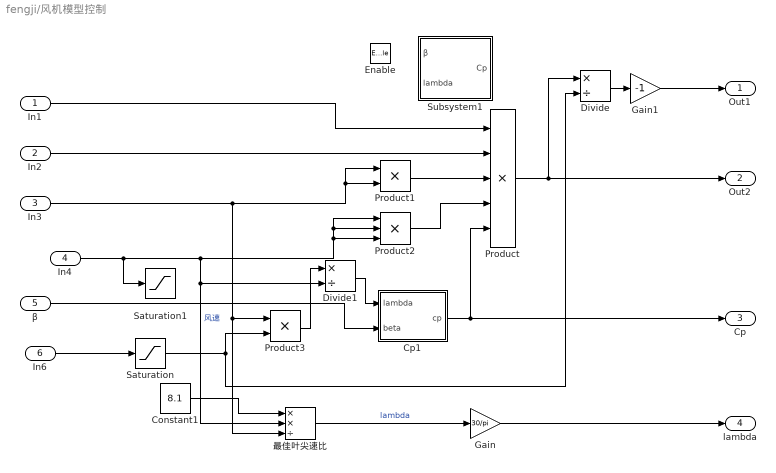
== system fengji/风机模型控制 ==
  In1 : Inport
  In2 : Inport  Port=2
  In3 : Inport  Port=3
  In4 : Inport  Port=4
  β : Inport  Port=5
  In6 : Inport  Port=6
  Enable : EnablePort
  Constant1 : Constant  Value=8.1
  Cp1 : Subsystem
  Divide : Product  Inputs=*/
  Divide1 : Product  Inputs=*/
  Gain : Gain  Gain=30/pi
  Gain1 : Gain  Gain=-1
  Product : Product  Inputs=5
  Product1 : Product
  Product2 : Product  Inputs=3
  Product3 : Product
  Saturation : Saturate  UpperLimit=1e6  LowerLimit=1e-6
  Saturation1 : Saturate  UpperLimit=1e6  LowerLimit=1e-6
  Subsystem1 : Subsystem
  最佳叶尖速比 : Product  Inputs=**/
  Out1 : Outport
  Out2 : Outport  Port=2
  Cp : Outport  Port=3
  lambda : Outport  Port=4
  wires:
  Product2/1 -> Product/4
  Divide/1 -> Gain1/1
  In3/1 -> Product3/1, 最佳叶尖速比/3, Product1/1, Product1/2
  Saturation/1 -> Divide/2, Product3/2
  Cp1/1(cp) -> Cp/1, Product/5
  Constant1/1 -> 最佳叶尖速比/1
  Product/1 -> Out2/1, Divide/1
  Product1/1 -> Product/3
  In4/1 -> Saturation1/1, Divide1/2, 最佳叶尖速比/2, Product2/3, Product2/2, Product2/1  "风速"
  In1/1 -> Product/1
  In6/1 -> Saturation/1
  Gain1/1 -> Out1/1
  In2/1 -> Product/2
  最佳叶尖速比/1 -> Gain/1  "lambda"
  β/1 -> Cp1/2(beta)
  Product3/1 -> Divide1/1
  Divide1/1 -> Cp1/1(lambda)
  Gain/1 -> lambda/1

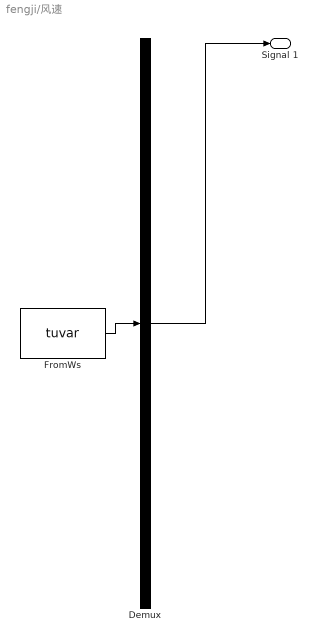
== system fengji/风速 ==
  Demux : Demux  Tag=STV Demux  Outputs=1
      settings: DisplayOption=none
  FromWs : FromWorkspace  Tag=STV FromWs  VariableName=tuvar
      SigBuilderData=|
      | common.afterFinalStr = 'Extrapolate'
      | common.sampleTime = 0
      | dataSet.timeRange = [0 3]
      | dataSet.name = 'Group 1'
      | sbobj.Groups.Name = 'Group 1'
      | sbobj.Groups.Signals.Name = 'Signal 1'
      | sbobj.Groups.Signals.XData = [0 1 1 3]
      | sbobj.Groups.Signals.YData = [8 8 12 12]
      | sbobj.Groups.TimeRange = [0 3]
  Signal 1 : Outport  Tag=STV Outport
  wires:
  Demux/1 -> Signal 1/1
  FromWs/1 -> Demux/1

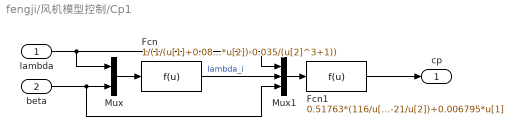
== system fengji/风机模型控制/Cp1 ==
  lambda : Inport
  beta : Inport  Port=2
  Fcn : Fcn  Expr=1/(1/(u[1]+0.08*u[2])-0.035/(u[2]^3+1))
  Fcn1 : Fcn  Expr=0.51763*(116/u[2]-0.4*u[3]-5)*exp(-21/u[2])+0.006795*u[1]
  Mux : Mux  Inputs=2
  Mux1 : Mux  Inputs=3
  cp : Outport  VectorParamsAs1DForOutWhenUnconnected=off
  wires:
  Mux/1 -> Fcn/1
  Mux1/1 -> Fcn1/1
  Fcn1/1 -> cp/1
  beta/1 -> Mux/2, Mux1/3
  lambda/1 -> Mux/1, Mux1/1
  Fcn/1 -> Mux1/2  "lambda_i"

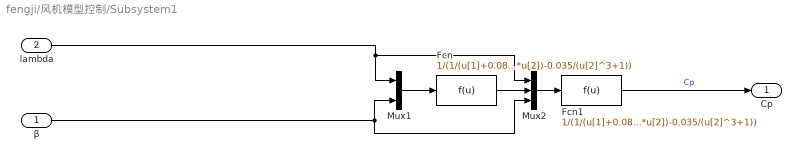
== system fengji/风机模型控制/Subsystem1 ==
  β : Inport
  lambda : Inport  Port=2
  Fcn : Fcn  Expr=1/(1/(u[1]+0.08*u[2])-0.035/(u[2]^3+1))
  Fcn1 : Fcn  Expr=1/(1/(u[1]+0.08*u[2])-0.035/(u[2]^3+1))
  Mux1 : Mux  Inputs=2
  Mux2 : Mux  Inputs=3
  Cp : Outport
  wires:
  β/1 -> Mux2/3, Mux1/2
  Fcn/1 -> Mux2/2
  Mux1/1 -> Fcn/1
  Mux2/1 -> Fcn1/1
  lambda/1 -> Mux2/1, Mux1/1
  Fcn1/1 -> Cp/1  "Cp"
